simulink model "controller_fault_injector"  (R2018b)
settings: Solver=FixedStepDiscrete  StartTime=0.0  StopTime=10.0  RelTol=1e-3
values from neighbouring files (symbols this model uses):
  EStop1_fi = int32(2^7)    [setup.m]
  EStop2_fi = int32(2^8)    [setup.m]
  EStop_fi = int32(2^6)    [setup.m]
  LevelControl_button1_fi = int32(2^4)    [setup.m]
  LevelControl_button2_fi = int32(2^5)    [setup.m]
  LevelControl_button_fi = int32(2^3)    [setup.m]
  Startup1_fi = int32(2^10)    [setup.m]
  Startup2_fi = int32(2^11)    [setup.m]
  Startup_fi = int32(2^9)    [setup.m]
  TempControl_button1_fi = int32(2^1)    [setup.m]
  TempControl_button2_fi = int32(2^2)    [setup.m]
  TempControl_button_fi = int32(2^0)    [setup.m]
  Thermocouple1_fi = int32(2^16)    [setup.m]
  Thermocouple2_fi = int32(2^17)    [setup.m]
  Thermocouple_fi = int32(2^15)    [setup.m]
  Thermocouple_fi_bitmask = uint16(0)    [setup.m]
  WaterLevelSensor1_fi = int32(2^13)    [setup.m]
  WaterLevelSensor2_fi = int32(2^14)    [setup.m]
  WaterLevelSensor_fi = int32(2^12)    [setup.m]
  WaterLevelSensor_fi_bitmask = uint16(128)    [setup.m]
libraries: library x18, simulink x2
settings Model: Creator=hiterd  LastModifiedBy=hiterd

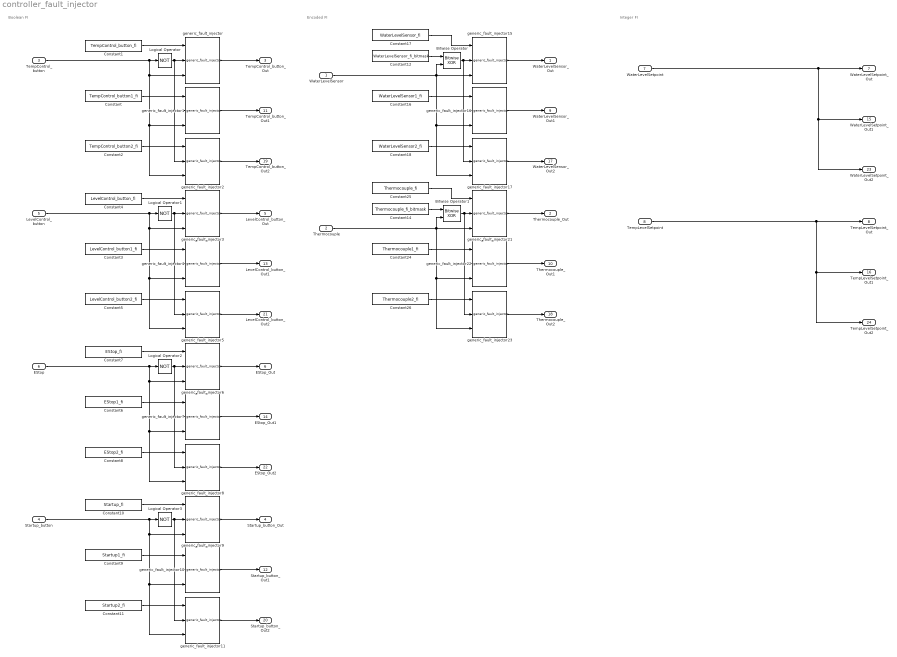
== system controller_fault_injector ==
  note: Encoded FI
  note: Boolean FI
  note: Integer FI
  WaterLevelSensor : Inport  OutDataTypeStr=uint16
  Thermocouple : Inport  Port=2  OutDataTypeStr=uint16
  TempControl_button : Inport  Port=3
  Startup_button : Inport  Port=4
  LevelControl_button : Inport  Port=5
  EStop : Inport  Port=6
  WaterLevelSetpoint : Inport  Port=7  OutDataTypeStr=uint16
  TempLevelSetpoint : Inport  Port=8  OutDataTypeStr=uint16
  Bitwise Operator : simulink/Logic and Bit Operations/Bitwise Operator  logicop=XOR  UseBitMask=off  NumInputPorts=2  BitMask=bin2dec('11011001')  BitMaskRealWorld=Stored Integer
  Bitwise Operator1 : simulink/Logic and Bit Operations/Bitwise Operator  logicop=XOR  UseBitMask=off  NumInputPorts=2  BitMask=bin2dec('11011001')  BitMaskRealWorld=Stored Integer
  Constant : Constant  Value=TempControl_button1_fi  SampleTime=-1
  Constant1 : Constant  Value=TempControl_button_fi  SampleTime=-1
  Constant10 : Constant  Value=Startup_fi  SampleTime=-1
  Constant11 : Constant  Value=Startup2_fi  SampleTime=-1
  Constant12 : Constant  Value=WaterLevelSensor_fi_bitmask  SampleTime=-1
  Constant14 : Constant  Value=Thermocouple_fi_bitmask  SampleTime=-1
  Constant16 : Constant  Value=WaterLevelSensor1_fi  SampleTime=-1
  Constant17 : Constant  Value=WaterLevelSensor_fi  SampleTime=-1
  Constant18 : Constant  Value=WaterLevelSensor2_fi  SampleTime=-1
  Constant2 : Constant  Value=TempControl_button2_fi  SampleTime=-1
  Constant24 : Constant  Value=Thermocouple1_fi  SampleTime=-1
  Constant25 : Constant  Value=Thermocouple_fi  SampleTime=-1
  Constant26 : Constant  Value=Thermocouple2_fi  SampleTime=-1
  Constant3 : Constant  Value=LevelControl_button1_fi  SampleTime=-1
  Constant4 : Constant  Value=LevelControl_button_fi  SampleTime=-1
  Constant5 : Constant  Value=LevelControl_button2_fi  SampleTime=-1
  Constant6 : Constant  Value=EStop1_fi  SampleTime=-1
  Constant7 : Constant  Value=EStop_fi  SampleTime=-1
  Constant8 : Constant  Value=EStop2_fi  SampleTime=-1
  Constant9 : Constant  Value=Startup1_fi  SampleTime=-1
  Logical Operator{,1..3} (4 alike) : Logic  Operator=NOT  Inputs=1  IconShape=distinctive  AllPortsSameDT=off  OutDataTypeStr=boolean
  generic_fault_injector{,1..11,15..17,21..23} (18 alike) : library/generic_fault_injector  SystemSampleTime=-1
  WaterLevelSensor_Out : Outport
  Thermocouple_Out : Outport  Port=2
  TempControl_button_Out : Outport  Port=3
  Startup_button_Out : Outport  Port=4
  LevelControl_button_Out : Outport  Port=5
  EStop_Out : Outport  Port=6
  WaterLevelSetpoint_Out : Outport  Port=7
  TempLevelSetpoint_Out : Outport  Port=8
  WaterLevelSensor_Out1 : Outport  Port=9
  Thermocouple_Out1 : Outport  Port=10
  TempControl_button_Out1 : Outport  Port=11
  Startup_button_Out1 : Outport  Port=12
  LevelControl_button_Out1 : Outport  Port=13
  EStop_Out1 : Outport  Port=14
  WaterLevelSetpoint_Out1 : Outport  Port=15
  TempLevelSetpoint_Out1 : Outport  Port=16
  WaterLevelSensor_Out2 : Outport  Port=17
  Thermocouple_Out2 : Outport  Port=18
  TempControl_button_Out2 : Outport  Port=19
  Startup_button_Out2 : Outport  Port=20
  LevelControl_button_Out2 : Outport  Port=21
  EStop_Out2 : Outport  Port=22
  WaterLevelSetpoint_Out2 : Outport  Port=23
  TempLevelSetpoint_Out2 : Outport  Port=24
  wires:
  Logical Operator/1 -> generic_fault_injector1/2, generic_fault_injector2/2, generic_fault_injector/2
  TempControl_button/1 -> generic_fault_injector1/3, generic_fault_injector2/3, generic_fault_injector/3, Logical Operator/1
  generic_fault_injector/1 -> TempControl_button_Out/1
  generic_fault_injector1/1 -> TempControl_button_Out1/1
  generic_fault_injector2/1 -> TempControl_button_Out2/1
  Constant/1 -> generic_fault_injector1/1
  Constant1/1 -> generic_fault_injector/1
  Constant2/1 -> generic_fault_injector2/1
  generic_fault_injector5/1 -> LevelControl_button_Out2/1
  Constant4/1 -> generic_fault_injector3/1
  generic_fault_injector4/1 -> LevelControl_button_Out1/1
  generic_fault_injector3/1 -> LevelControl_button_Out/1
  Constant5/1 -> generic_fault_injector5/1
  Constant3/1 -> generic_fault_injector4/1
  LevelControl_button/1 -> generic_fault_injector4/3, generic_fault_injector5/3, generic_fault_injector3/3, Logical Operator1/1
  Logical Operator1/1 -> generic_fault_injector4/2, generic_fault_injector5/2, generic_fault_injector3/2
  generic_fault_injector6/1 -> EStop_Out/1
  generic_fault_injector7/1 -> EStop_Out1/1
  Constant7/1 -> generic_fault_injector6/1
  Logical Operator2/1 -> generic_fault_injector7/2, generic_fault_injector8/2, generic_fault_injector6/2
  generic_fault_injector8/1 -> EStop_Out2/1
  EStop/1 -> generic_fault_injector7/3, generic_fault_injector8/3, generic_fault_injector6/3, Logical Operator2/1
  Constant6/1 -> generic_fault_injector7/1
  Constant8/1 -> generic_fault_injector8/1
  generic_fault_injector11/1 -> Startup_button_Out2/1
  Startup_button/1 -> generic_fault_injector10/3, generic_fault_injector11/3, generic_fault_injector9/3, Logical Operator3/1
  generic_fault_injector9/1 -> Startup_button_Out/1
  Constant9/1 -> generic_fault_injector10/1
  Constant10/1 -> generic_fault_injector9/1
  Constant11/1 -> generic_fault_injector11/1
  generic_fault_injector10/1 -> Startup_button_Out1/1
  Logical Operator3/1 -> generic_fault_injector10/2, generic_fault_injector11/2, generic_fault_injector9/2
  Constant18/1 -> generic_fault_injector17/1
  Constant17/1 -> generic_fault_injector15/1
  Constant16/1 -> generic_fault_injector16/1
  generic_fault_injector15/1 -> WaterLevelSensor_Out/1
  generic_fault_injector17/1 -> WaterLevelSensor_Out2/1
  WaterLevelSensor/1 -> Bitwise Operator/2, generic_fault_injector15/3, generic_fault_injector16/3, generic_fault_injector17/3
  generic_fault_injector16/1 -> WaterLevelSensor_Out1/1
  Constant26/1 -> generic_fault_injector23/1
  Constant25/1 -> generic_fault_injector21/1
  Constant24/1 -> generic_fault_injector22/1
  generic_fault_injector21/1 -> Thermocouple_Out/1
  Bitwise Operator1/1 -> generic_fault_injector23/2, generic_fault_injector22/2, generic_fault_injector21/2
  generic_fault_injector23/1 -> Thermocouple_Out2/1
  Thermocouple/1 -> Bitwise Operator1/2, generic_fault_injector22/3, generic_fault_injector23/3, generic_fault_injector21/3
  generic_fault_injector22/1 -> Thermocouple_Out1/1
  WaterLevelSetpoint/1 -> WaterLevelSetpoint_Out2/1, WaterLevelSetpoint_Out1/1, WaterLevelSetpoint_Out/1
  TempLevelSetpoint/1 -> TempLevelSetpoint_Out2/1, TempLevelSetpoint_Out1/1, TempLevelSetpoint_Out/1
  Constant12/1 -> Bitwise Operator/1
  Bitwise Operator/1 -> generic_fault_injector17/2, generic_fault_injector16/2, generic_fault_injector15/2
  Constant14/1 -> Bitwise Operator1/1
